simulink library "csu_egd_engine_disturbance_lib"  (R2014b)
settings: Solver=ode45  StartTime=0.0  StopTime=10.0  RelTol=1e-3
values from neighbouring files (symbols this model uses):
  csc_gdn_prep_main_thruster_orientation = psp_thruster25_orientation    [csu_egd_engine_disturbance_prep.m]
  csc_gdn_prep_main_thruster_position = psp_thruster25_position    [csu_egd_engine_disturbance_prep.m]
undefined symbols (not defined in the file or in its folder): csc_gdn_prep_thrust_available
libraries: util_info_lib x1, util_common_lib x1
settings Model: Creator=ianmga  LastModifiedBy=mstewart

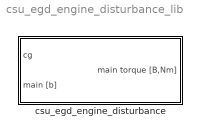
== system csu_egd_engine_disturbance_lib ==
  csu_egd_engine_disturbance : Subsystem

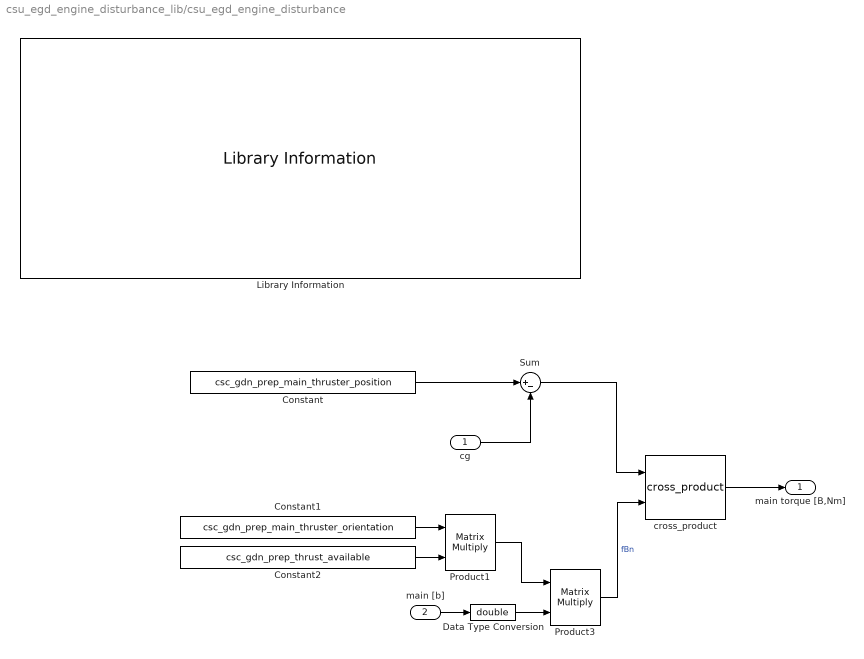
== system csu_egd_engine_disturbance_lib/csu_egd_engine_disturbance ==
  cg : Inport
  main [b] : Inport  Port=2
  Constant : Constant  Value=csc_gdn_prep_main_thruster_position
  Constant1 : Constant  Value=csc_gdn_prep_main_thruster_orientation
  Constant2 : Constant  Value=csc_gdn_prep_thrust_available
  Data Type Conversion : DataTypeConversion  OutDataTypeStr=double
  Library Information : util_info_lib/Library Information  owner='NONE'
  Product1 : Product  Multiplication=Matrix(*)  RndMeth=Zero
  Product3 : Product  Multiplication=Matrix(*)  RndMeth=Zero
  Sum : Sum  Inputs=|+-
  cross_product : util_common_lib/cross_product  SystemSampleTime=-1
  main torque [B,Nm] : Outport
  wires:
  Data Type Conversion/1 -> Product3/2
  cross_product/1 -> main torque [B,Nm]/1
  Sum/1 -> cross_product/1
  Constant/1 -> Sum/1
  Product3/1 -> cross_product/2  "fBn"
  main [b]/1 -> Data Type Conversion/1
  cg/1 -> Sum/2
  Constant2/1 -> Product1/2
  Constant1/1 -> Product1/1
  Product1/1 -> Product3/1
